simulink model "Second_Order_Nonlinear_RLC_Systems"  (R2021b)
settings: Solver=ode5  StartTime=0.0  StopTime=30  RelTol=1e-3
values from neighbouring files (symbols this model uses):
  C = 1    [Sliding_Mode_Controller.m]
  eta = 0.1    [Sliding_Mode_Controller.m]
  L = 1    [Sliding_Mode_Controller.m]
  lambda = 20    [Sliding_Mode_Controller.m]
  R = 1    [Sliding_Mode_Controller.m]
  su = 0.5    [Sliding_Mode_Controller.m]
settings Model: Creator=Nambi  LastModifiedBy=Nambi
settings DataIOCC: ReturnWorkspaceOutputs=off

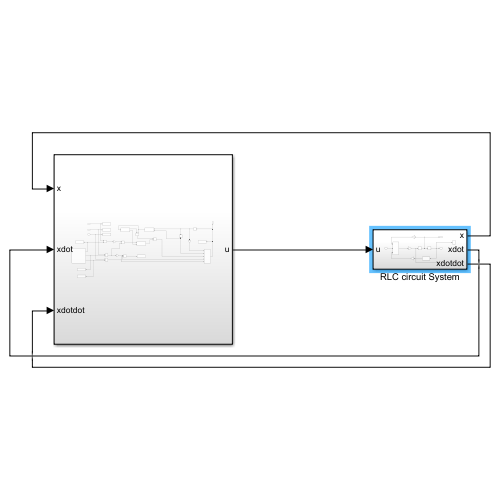
[thumbnail: Simulink's stored preview of the top-level diagram]
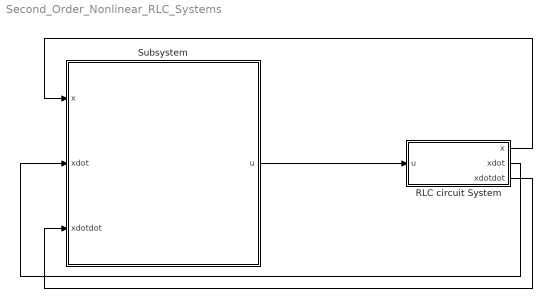
== system Second_Order_Nonlinear_RLC_Systems ==
  RLC circuit System : Subsystem
  Subsystem : Subsystem
  wires:
  Subsystem/1(u) -> RLC circuit System/1(u)
  RLC circuit System/1(x) -> Subsystem/1(x)
  RLC circuit System/3(xdotdot) -> Subsystem/3(xdotdot)
  RLC circuit System/2(xdot) -> Subsystem/2(xdot)

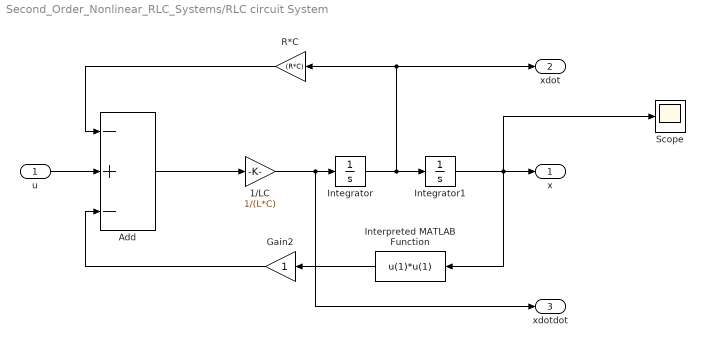
== system Second_Order_Nonlinear_RLC_Systems/RLC circuit System ==
  u : Inport
  1/LC : Gain  Gain=1/(L*C)
  Add : Sum  Inputs=-+-
  Gain2 : Gain
  Integrator : Integrator  InitialCondition=pi/2
  Integrator1 : Integrator
  Interpreted MATLAB Function : MATLABFcn  MATLABFcn=u(1)*u(1)
  R*C : Gain  Gain=(R*C)
  Scope : Scope
  x : Outport
  xdot : Outport  Port=2
  xdotdot : Outport  Port=3
  wires:
  R*C/1 -> Add/1
  u/1 -> Add/2
  Gain2/1 -> Add/3
  Integrator1/1 -> Interpreted MATLAB Function/1, Scope/1, x/1
  Add/1 -> 1/LC/1
  1/LC/1 -> xdotdot/1, Integrator/1
  Integrator/1 -> xdot/1, R*C/1, Integrator1/1
  Interpreted MATLAB Function/1 -> Gain2/1

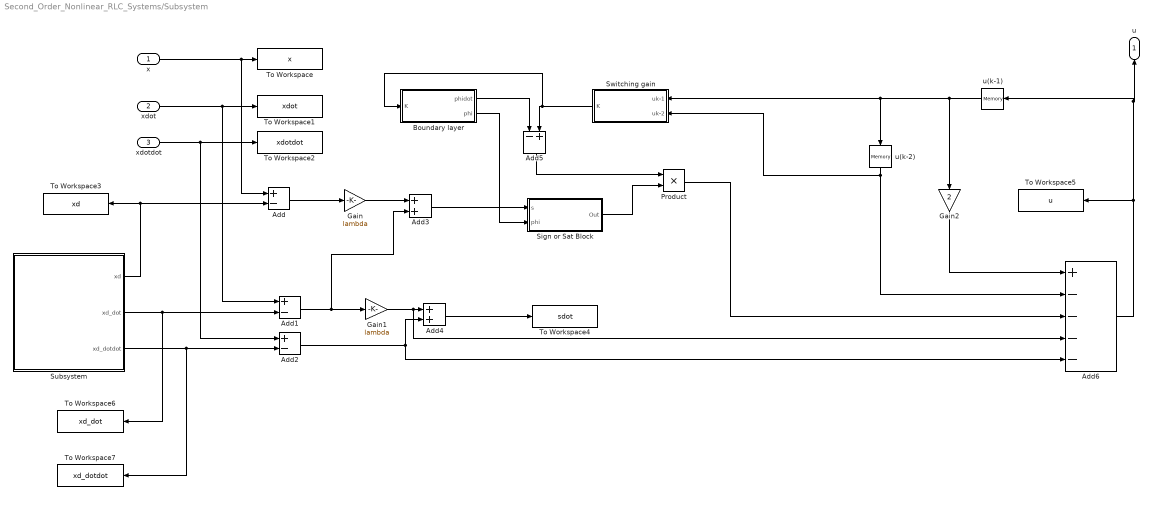
== system Second_Order_Nonlinear_RLC_Systems/Subsystem ==
  x : Inport
  xdot : Inport  Port=2
  xdotdot : Inport  Port=3
  Add : Sum  Inputs=+-
  Add1 : Sum  Inputs=+-
  Add2 : Sum  Inputs=+-
  Add3 : Sum
  Add4 : Sum
  Add5 : Sum  Inputs=-+
  Add6 : Sum  Inputs=+----
  Boundary layer : Subsystem
  Gain : Gain  Gain=lambda
  Gain1 : Gain  Gain=lambda
  Gain2 : Gain  Gain=2
  Product : Product
  Sign or Sat Block : Subsystem
  Subsystem : Subsystem
  Switching gain : Subsystem
  To Workspace : ToWorkspace  VariableName=x  SampleTime=-1
  To Workspace1 : ToWorkspace  VariableName=xdot  SampleTime=-1
  To Workspace2 : ToWorkspace  VariableName=xdotdot  SampleTime=-1
  To Workspace3 : ToWorkspace  VariableName=xd  SampleTime=-1
  To Workspace4 : ToWorkspace  VariableName=sdot  SampleTime=-1
  To Workspace5 : ToWorkspace  VariableName=u  SampleTime=-1
  To Workspace6 : ToWorkspace  VariableName=xd_dot  SampleTime=-1
  To Workspace7 : ToWorkspace  VariableName=xd_dotdot  SampleTime=-1
  u(k-1) : Memory
  u(k-2) : Memory
  u : Outport
  wires:
  Subsystem/1(xd) -> To Workspace3/1, Add/2
  Boundary layer/1(phidot) -> Add5/1
  u(k-2)/1 -> Add6/2, Switching gain/2(uk-2)
  u(k-1)/1 -> Switching gain/1(uk-1), u(k-2)/1, Gain2/1
  Gain2/1 -> Add6/1
  Boundary layer/2(phi) -> Sign or Sat Block/2(phi)
  Sign or Sat Block/1(Out) -> Product/2
  Add3/1 -> Sign or Sat Block/1(s)
  Gain1/1 -> Add6/4, Add4/1
  xdotdot/1 -> Add2/1, To Workspace2/1
  Product/1 -> Add6/3
  Gain/1 -> Add3/1
  Subsystem/3(xd_dotdot) -> To Workspace7/1, Add2/2
  Add2/1 -> Add6/5, Add4/2
  xdot/1 -> Add1/1, To Workspace1/1
  Add1/1 -> Add3/2, Gain1/1
  Add/1 -> Gain/1
  Subsystem/2(xd_dot) -> To Workspace6/1, Add1/2
  Add4/1 -> To Workspace4/1
  Add5/1 -> Product/1
  Switching gain/1(K) -> Boundary layer/1(K), Add5/2
  x/1 -> Add/1, To Workspace/1
  Add6/1 -> To Workspace5/1, u/1, u(k-1)/1

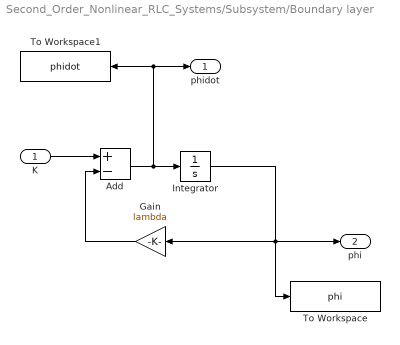
== system Second_Order_Nonlinear_RLC_Systems/Subsystem/Boundary layer ==
  K : Inport
  Add : Sum  Inputs=+-
  Gain : Gain  Gain=lambda
  Integrator : Integrator
  To Workspace : ToWorkspace  VariableName=phi  SampleTime=-1
  To Workspace1 : ToWorkspace  VariableName=phidot  SampleTime=-1
  phidot : Outport
  phi : Outport  Port=2
  wires:
  K/1 -> Add/1
  Gain/1 -> Add/2
  Add/1 -> phidot/1, To Workspace1/1, Integrator/1
  Integrator/1 -> To Workspace/1, phi/1, Gain/1

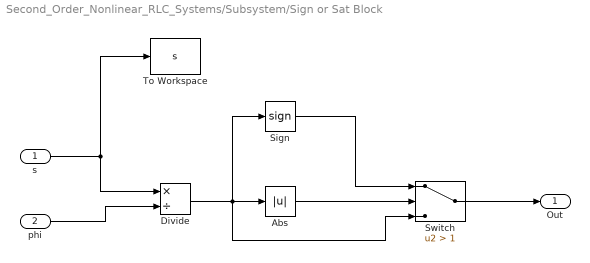
== system Second_Order_Nonlinear_RLC_Systems/Subsystem/Sign or Sat Block ==
  s : Inport
  phi : Inport  Port=2
  "Abs " : Abs
  Divide : Product  Inputs=*/
  "Sign " : Signum
  Switch : Switch  Criteria=u2 > Threshold  Threshold=1
  To Workspace : ToWorkspace  VariableName=s  SampleTime=-1
  Out : Outport
  wires:
  Divide/1 -> Switch/3, "Sign "/1, "Abs "/1
  "Abs "/1 -> Switch/2
  "Sign "/1 -> Switch/1
  Switch/1 -> Out/1
  s/1 -> Divide/1, To Workspace/1
  phi/1 -> Divide/2

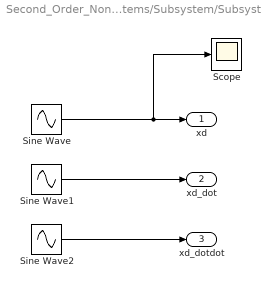
== system Second_Order_Nonlinear_RLC_Systems/Subsystem/Subsystem ==
  Scope : Scope
  Sine Wave : Sin  Frequency=pi/2  SampleTime=0.0001
  Sine Wave1 : Sin  Amplitude=1*pi/2  Frequency=pi/2  Phase=pi/2  SampleTime=0.0001
  Sine Wave2 : Sin  Amplitude=-1*pi/2*pi/2  Frequency=pi/2  SampleTime=0.0001
  xd : Outport
  xd_dot : Outport  Port=2
  xd_dotdot : Outport  Port=3
  wires:
  Sine Wave/1 -> Scope/1, xd/1
  Sine Wave1/1 -> xd_dot/1
  Sine Wave2/1 -> xd_dotdot/1

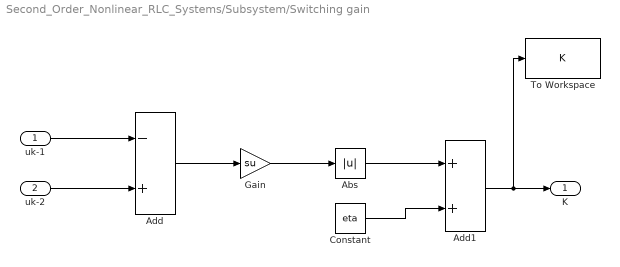
== system Second_Order_Nonlinear_RLC_Systems/Subsystem/Switching gain ==
  uk-1 : Inport
  uk-2 : Inport  Port=2
  Abs : Abs
  Add : Sum  Inputs=-+
  Add1 : Sum
  Constant : Constant  Value=eta
  Gain : Gain  Gain=su
  To Workspace : ToWorkspace  VariableName=K  SampleTime=-1
  K : Outport
  wires:
  uk-1/1 -> Add/1
  uk-2/1 -> Add/2
  Add/1 -> Gain/1
  Gain/1 -> Abs/1
  Abs/1 -> Add1/1
  Constant/1 -> Add1/2
  Add1/1 -> To Workspace/1, K/1
